simulink library "powerlib_models"  (Simulink 6.0)
settings: Solver=ode45  SolverMode=SingleTasking  StartTime=0.0  StopTime=10.0  RelTol=1e-3
values from neighbouring files (symbols this model uses):
  Ts = get(handles.edit1,'string')    [powergui.m]
undefined symbols (not defined in the file or in its folder): A, a0, a1, a2, a3, a4, a5, Ac, Amplitude, Amplitudes, B, BaseCurrent, BaseFlux, Bc, C, Capacitance, Cc, Columns, ConnectionType, Cs, ctrl, current, Current, damp, Dc, Dd, DiscIntNeverNeededParam, dref, dwo, exc, excAxis, F, Flux, fnom, Frequency, FreqVps, Gain1, gate, GH, GHd, GI, GId, GL, GLd, H, HarmonicGeneration, HT, hyd, I1_init, ib, ib2, Id1o, Inductance, InitialFlux, InitialSlope, io, Iq1o, isfinite, j, J ... (+138)
libraries: powerlib_models x32, powerlib_extras x4
(part 9 of 11)

== system powerlib_models/Phasors/simplified_sync_mach/Idq1 Idq2 Pe  ==
  note: I2= -V2/Z
  note: I1= (E-V1)/Z
  note: V1= 1/3(Vab -a^2*Vbc)
  note: V2= 1/3(Vab -a*Vbc)
  Vab Vbc cmplx : Inport  Port=1  LatchInput=off
  e : Inport  Port=2  LatchInput=off
  delta : Inport  Port=3  LatchInput=off
  (a^2)/3 : Gain  Gain=1/3*exp(-j*2*pi/3)  SaturateOnIntegerOverflow=on
  -1 : Gain  Gain=-1  SaturateOnIntegerOverflow=on
  1/Z1 : Gain  Gain=1/(R+j*L)  SaturateOnIntegerOverflow=on
  Complex to Real-Imag : ComplexToRealImag  Output=Real
  Complex to Real-Imag1 : ComplexToRealImag
  Complex to Real-Imag2 : ComplexToRealImag
  Complex to Real-Imag3 : ComplexToRealImag
  Demux : Demux  Outputs=2
  Gain : Gain  Gain=1/3  SaturateOnIntegerOverflow=on
  Gain1 : Gain  Gain=1/3  SaturateOnIntegerOverflow=on
  Magnitude-Angle to Complex1 : MagnitudeAngleToComplex
  Mux1 : Mux  Inputs=2
  Mux2 : Mux  Inputs=2
  Product : Product  SaturateOnIntegerOverflow=on  InputSameDT=on
  Real-Imag to Complex : RealImagToComplex
  Sum1 : Sum  Inputs=-+  SaturateOnIntegerOverflow=on  InputSameDT=on
  Sum3 : Sum  Inputs=+-  SaturateOnIntegerOverflow=on  InputSameDT=on
  Sum4 : Sum  Inputs=+-  SaturateOnIntegerOverflow=on  InputSameDT=on
  Vdq1->Idq1 : Subsystem
  Vdq2->Idq2 : Subsystem
  a/3 : Gain  Gain=1/3*exp(j*2*pi/3)  SaturateOnIntegerOverflow=on
  conj : Gain  Gain=-1  SaturateOnIntegerOverflow=on
  Pe : Outport
  Idq1 : Outport  Port=2
  Idq2 : Outport  Port=3
  wires:
  conj/1 -> Real-Imag to Complex/2
  Complex to Real-Imag1/2 -> conj/1
  Complex to Real-Imag1/1 -> Real-Imag to Complex/1
  Real-Imag to Complex/1 -> Product/2
  Magnitude-Angle to Complex1/1 -> Complex to Real-Imag1/1, Sum1/2  "E"
  Complex to Real-Imag/1 -> Pe/1
  Product/1 -> Complex to Real-Imag/1
  1/Z1/1 -> Product/1
  Sum1/1 -> 1/Z1/1, Complex to Real-Imag2/1  "U1=E1-V1"
  Sum3/1 -> Sum1/1  "V1"
  delta/1 -> Magnitude-Angle to Complex1/2
  e/1 -> Magnitude-Angle to Complex1/1
  Demux/1 -> Gain1/1, Gain/1
  a/3/1 -> Sum4/2
  Gain1/1 -> Sum4/1
  Vab Vbc cmplx/1 -> Demux/1
  Gain/1 -> Sum3/1
  Demux/2 -> a/3/1, (a^2)/3/1
  (a^2)/3/1 -> Sum3/2
  Sum4/1 -> -1/1  "V2"
  -1/1 -> Complex to Real-Imag3/1  "-V2"
  Complex to Real-Imag2/1 -> Mux1/1
  Complex to Real-Imag2/2 -> Mux1/2
  Complex to Real-Imag3/1 -> Mux2/1
  Complex to Real-Imag3/2 -> Mux2/2
  Mux1/1 -> Vdq1->Idq1/1(In1)
  Mux2/1 -> Vdq2->Idq2/1(In1)
  Vdq1->Idq1/1(Out1) -> Idq1/1
  Vdq2->Idq2/1(Out1) -> Idq2/1

== system powerlib_models/Phasors/simplified_sync_mach/LL2LN ==
  note: Vcn= -Van - Vbn
  note: Vbn=(Vbc - Vab)/3
  note: Van=(2*Vab+Vbc))/3
  Vab_bc : Inport  Port=1  LatchInput=off
  1/3 : Gain  Gain=1/3  SaturateOnIntegerOverflow=on
  2 : Gain  Gain=2  SaturateOnIntegerOverflow=on
  Demux : Demux  Outputs=2
  Mux2 : Mux  Inputs=3
  Sum1 : Sum  SaturateOnIntegerOverflow=on  InputSameDT=on
  Sum2 : Sum  Inputs=+-  SaturateOnIntegerOverflow=on  InputSameDT=on
  Sum6 : Sum  Orientation=down  Inputs=--  SaturateOnIntegerOverflow=on  InputSameDT=on
  Vabc_n : Outport
  wires:
  Demux/2 -> Sum2/1, Sum1/2
  2/1 -> Sum1/1
  Demux/1 -> Sum2/2, 2/1
  1/3/1 -> Demux/1
  Mux2/1 -> Vabc_n/1
  Vab_bc/1 -> 1/3/1
  Sum1/1 -> Sum6/2, Mux2/1  "Van"
  Sum2/1 -> Sum6/1, Mux2/2  "Vbn"
  Sum6/1 -> Mux2/3

== system powerlib_models/Phasors/simplified_sync_mach/Phasors Ia Ib ==
  note: Ib= a^2*I1 + a*I2
  note: Ia= I1 + I2
  Idq1 : Inport  Port=1  LatchInput=off
  Idq2 : Inport  Port=2  LatchInput=off
  Demux : Demux  Outputs=2
  Demux1 : Demux  Outputs=2
  Mux1 : Mux  Inputs=2
  Mux2 : Mux  Inputs=[2 1]
  Real-Imag to Complex : RealImagToComplex
  Real-Imag to Complex2 : RealImagToComplex
  Sum : Sum  Orientation=down  Inputs=1  SaturateOnIntegerOverflow=on  InputSameDT=on
  Sum1 : Sum  SaturateOnIntegerOverflow=on  InputSameDT=on
  Sum3 : Sum  SaturateOnIntegerOverflow=on  InputSameDT=on
  a : Gain  Gain=exp(j*2*pi/3)  SaturateOnIntegerOverflow=on
  a^2 : Gain  Gain=exp(-j*2*pi/3)  SaturateOnIntegerOverflow=on
  inv : Gain  Gain=-1  SaturateOnIntegerOverflow=on
  Iabc cmplx : Outport
  Iab cmplx : Outport  Port=2
  wires:
  Real-Imag to Complex2/1 -> a/1, Sum3/2  "I2"
  Idq2/1 -> Demux1/1
  Demux1/2 -> Real-Imag to Complex2/2
  Demux1/1 -> Real-Imag to Complex2/1
  Real-Imag to Complex/1 -> Sum3/1, a^2/1  "I1"
  Mux2/1 -> Iabc cmplx/1
  inv/1 -> Mux2/2  "ic"
  Sum/1 -> inv/1
  Mux1/1 -> Sum/1, Mux2/1, Iab cmplx/1  "ia ib"
  Demux/2 -> Real-Imag to Complex/2
  Demux/1 -> Real-Imag to Complex/1
  Idq1/1 -> Demux/1
  Sum1/1 -> Mux1/2
  Sum3/1 -> Mux1/1
  a/1 -> Sum1/2
  a^2/1 -> Sum1/1

== system powerlib_models/Phasors/simplified_sync_mach/Subsystem ==
  i : Inport  Port=1  LatchInput=off
  v : Inport  Port=2  LatchInput=off
  e : Inport  Port=3  LatchInput=off
  theta : Inport  Port=4  LatchInput=off
  wm : Inport  Port=5  LatchInput=off
  Pe : Inport  Port=6  LatchInput=off
  Gain : Gain  Gain=[ ib2*ones(3,1); Vb3*ones(6,1); 1; Nb; Pb ]  SaturateOnIntegerOverflow=on
  Mux : Mux  Inputs=[ 3 3 3 1 1 1 ]
  * : Outport  InitialOutput=0
  wires:
  Gain/1 -> */1
  Mux/1 -> Gain/1
  Pe/1 -> Mux/6
  wm/1 -> Mux/5
  theta/1 -> Mux/4
  e/1 -> Mux/3
  v/1 -> Mux/2
  i/1 -> Mux/1

== system powerlib_models/Phasors/synchronous_machine/Delta angle ==
  Vq : Inport  Port=1  PortDimensions=1  LatchInput=off
  Vd : Inport  Port=2  PortDimensions=1  LatchInput=off
  Cartesian to Polar : Subsystem
      mask Type: Cart2Polar
      mask Description:
      | Transformation from cartesian to polar coordinates.
      | [x, y] -> [r, theta]
      | 
      | r = sqrt(x^2 + y^2);
      | theta = atan(y/x);
      mask Help: Unmask this block for more help.
      mask Display: plot(0,0,100,100,[24,20,15,20,20],[85,95,85,95,20],[80,20,95,85,95,85],[70,20,20,15,20,24],[56,56,55,52,50,46],[20,26,31,35,38,42])
  Radians to Degrees : Subsystem
      mask Type: RadiansToDegrees
      mask Description:
      | Conversion from Radians to Degrees.
      | 
      | D=180/pi*R
      mask Help: This block converts from Radians to Degrees.
      mask Display: disp('R2D')
  Terminator2 : Terminator
  delta : Outport
  wires:
  Vd/1 -> Cartesian to Polar/2(y)
  Radians to Degrees/1(Degrees out) -> delta/1  "delta"
  Vq/1 -> Cartesian to Polar/1(x)
  Cartesian to Polar/1(r) -> Terminator2/1
  Cartesian to Polar/2(theta) -> Radians to Degrees/1(Radians in)

== system powerlib_models/Phasors/synchronous_machine/PQ ==
  note: P = Vd*Id + Vq*Iq
  note: Q = Vq*Id-Vd*Iq
  note: PQ Measurement:
  Vq : Inport  Port=1  PortDimensions=1  LatchInput=off
  Vd : Inport  Port=2  PortDimensions=1  LatchInput=off
  Iq : Inport  Port=3  PortDimensions=2  LatchInput=off
  Demux1 : Demux  Outputs=[1,1]
  Gain : Gain  Gain=Gain1  SaturateOnIntegerOverflow=on
  Gain1 : Gain  Gain=Gain1  SaturateOnIntegerOverflow=on
  Product{2..5} (4 alike) : Product  SaturateOnIntegerOverflow=on  InputSameDT=on
  Sum : Sum  SaturateOnIntegerOverflow=on  InputSameDT=on
  Sum1 : Sum  Inputs=+-  SaturateOnIntegerOverflow=on  InputSameDT=on
  Peo : Outport
  Qeo : Outport  Port=2
  wires:
  Demux1/1 -> Product5/2, Product2/2
  Iq/1 -> Demux1/1
  Gain1/1 -> Qeo/1
  Gain/1 -> Peo/1
  Product2/1 -> Sum/1
  Product3/1 -> Sum/2
  Product4/1 -> Sum1/1
  Product5/1 -> Sum1/2
  Sum/1 -> Gain/1  "Peo"
  Sum1/1 -> Gain1/1  "Qeo"
  Vd/1 -> Product3/1, Product5/1
  Vq/1 -> Product2/1, Product4/1
  Demux1/2 -> Product3/2, Product4/2

== system powerlib_models/Phasors/synchronous_machine/Phasors Ia Ib ==
  note: add angle d_theta
  note: Ib= a^2*I1 + a*I2
  note: Ia= I1 + I2
  Idq1 : Inport  Port=1  LatchInput=off
  d_theta : Inport  Port=2  LatchInput=off
  I2_cmplx : Inport  Port=3  LatchInput=off
  Demux : Demux  Outputs=2
  Gain2 : Gain  Gain=j  SaturateOnIntegerOverflow=on
  Math Function : Math  SaturateOnIntegerOverflow=on
  Mux1 : Mux  Inputs=2
  Mux2 : Mux  Inputs=[2 1]
  Product : Product  SaturateOnIntegerOverflow=on  InputSameDT=on
  Real-Imag to Complex : RealImagToComplex
  Sum : Sum  Orientation=down  Inputs=1  SaturateOnIntegerOverflow=on  InputSameDT=on
  Sum1 : Sum  SaturateOnIntegerOverflow=on  InputSameDT=on
  Sum3 : Sum  SaturateOnIntegerOverflow=on  InputSameDT=on
  a : Gain  Gain=exp(j*2*pi/3)  SaturateOnIntegerOverflow=on
  a^2 : Gain  Gain=exp(-j*2*pi/3)  SaturateOnIntegerOverflow=on
  inv : Gain  Gain=-1  SaturateOnIntegerOverflow=on
  Ia Ib cmplx : Outport
  Iabc cmplx : Outport  Port=2
  wires:
  d_theta/1 -> Gain2/1
  Real-Imag to Complex/1 -> Product/1  "I1 machine"
  Math Function/1 -> Product/2
  Gain2/1 -> Math Function/1
  Mux2/1 -> Iabc cmplx/1
  inv/1 -> Mux2/2  "ic"
  Sum/1 -> inv/1
  Mux1/1 -> Mux2/1, Ia Ib cmplx/1, Sum/1  "ia ib"
  Demux/2 -> Real-Imag to Complex/2
  Demux/1 -> Real-Imag to Complex/1
  Idq1/1 -> Demux/1
  Product/1 -> Sum3/1, a^2/1  "I1"
  Sum1/1 -> Mux1/2
  Sum3/1 -> Mux1/1
  a/1 -> Sum1/2
  a^2/1 -> Sum1/1
  I2_cmplx/1 -> Sum3/2, a/1  "I2"

== system powerlib_models/Phasors/synchronous_machine/Subsystem ==
  Vf : Inport  Port=1  LatchInput=off
  Constant : Constant  Value=excAxis
  Ground2 : Ground
  Switch : Switch  Threshold=1.5  InputSameDT=on
  Switch1 : Switch  Threshold=1.5  InputSameDT=on
  Vkq1 : Outport
  Vfd : Outport  Port=2
  wires:
  Switch/1 -> Vkq1/1
  Switch1/1 -> Vfd/1
  Constant/1 -> Switch1/2, Switch/2
  Vf/1 -> Switch/1, Switch1/3
  Ground2/1 -> Switch/3, Switch1/1

== system powerlib_models/Phasors/synchronous_machine/Vd1 Vq1, I2  ==
  note: Subtract angle d_theta
  note: V2= 1/3(Vab -a*Vbc)
  note: V1= 1/3(Vab -a^2*Vbc)
  Vab Vbc cmplx : Inport  Port=1  LatchInput=off
  d_theta : Inport  Port=2  LatchInput=off
  (a^2)/3 : Gain  Gain=1/3*exp(-j*2*pi/3)  SaturateOnIntegerOverflow=on
  Complex to Real-Imag1 : ComplexToRealImag
  Complex to Real-Imag2 : ComplexToRealImag
  Demux : Demux  Outputs=2
  Gain : Gain  Gain=1/3  SaturateOnIntegerOverflow=on
  Gain1 : Gain  Gain=1/3  SaturateOnIntegerOverflow=on
  Gain2 : Gain  Gain=-j  SaturateOnIntegerOverflow=on
  Math Function : Math  SaturateOnIntegerOverflow=on
  Mux2 : Mux  Inputs=2
  Product : Product  SaturateOnIntegerOverflow=on  InputSameDT=on
  Sum3 : Sum  Inputs=+-  SaturateOnIntegerOverflow=on  InputSameDT=on
  Sum4 : Sum  Inputs=+-  SaturateOnIntegerOverflow=on  InputSameDT=on
  Vdq2->Idq2 : Subsystem
  a/3 : Gain  Gain=1/3*exp(j*2*pi/3)  SaturateOnIntegerOverflow=on
  Vd : Outport
  Vq : Outport  Port=2
  I2_cmplx : Outport  Port=3
  wires:
  Math Function/1 -> Product/2
  Product/1 -> Complex to Real-Imag1/1
  Gain2/1 -> Math Function/1
  Sum4/1 -> Complex to Real-Imag2/1  "V2"
  (a^2)/3/1 -> Sum3/2
  Demux/2 -> (a^2)/3/1, a/3/1
  Complex to Real-Imag1/1 -> Vd/1
  Complex to Real-Imag1/2 -> Vq/1
  Sum3/1 -> Product/1  "V1"
  d_theta/1 -> Gain2/1
  Gain/1 -> Sum3/1
  Vab Vbc cmplx/1 -> Demux/1
  Gain1/1 -> Sum4/1
  a/3/1 -> Sum4/2
  Demux/1 -> Gain/1, Gain1/1
  Complex to Real-Imag2/1 -> Mux2/1
  Complex to Real-Imag2/2 -> Mux2/2
  Mux2/1 -> Vdq2->Idq2/1(V2_dq)
  Vdq2->Idq2/1(I2_cmplx) -> I2_cmplx/1

== system powerlib_models/Phasors/synchronous_machine/currents and mutual fluxes ==
  note: This subsystem computes the mutual fluxes phimd
      | and phimq and all direct and quadrature axis
      | currents in the model.
  phiq : Inport  Port=1  LatchInput=off
  phikq2 : Inport  Port=2  LatchInput=off
  phid : Inport  Port=3  LatchInput=off
  phifd : Inport  Port=4  LatchInput=off
  phikq1 : Inport  Port=5  LatchInput=off
  phikd : Inport  Port=6  LatchInput=off
  -1_Ll : Gain  Gain=-1/Ll  SaturateOnIntegerOverflow=on
  "-1_Ll " : Gain  Gain=-1/Ll  SaturateOnIntegerOverflow=on
  1_Llfd : Gain  Gain=1/Llfd  SaturateOnIntegerOverflow=on
  1_Llkd : Gain  Gain=1/Llkd  SaturateOnIntegerOverflow=on
  1_Llkq1 : Gain  Gain=1/Llkq1  SaturateOnIntegerOverflow=on
  1_Llkq2 : Gain  Gain=1/Llkq2  SaturateOnIntegerOverflow=on
  Lad_Ll : Gain  Gain=Lad/Ll  SaturateOnIntegerOverflow=on
  Lad_Llfd : Gain  Gain=Lad/Llfd  SaturateOnIntegerOverflow=on
  Lad_Llkd : Gain  Gain=Lad/Llkd  SaturateOnIntegerOverflow=on
  Laq_Ll : Gain  Gain=Laq/Ll  SaturateOnIntegerOverflow=on
  Laq_Llkq1 : Gain  Gain=Laq/Llkq1  SaturateOnIntegerOverflow=on
  Laq_Llkq2 : Gain  Gain=Laq/Llkq2  SaturateOnIntegerOverflow=on
  Mux1 : Mux  Inputs=2
  Mux3 : Mux  Inputs=[2 1 1 1 1 1 1]
  Saturation : Subsystem
  Sum{17..22} (6 alike) : Sum  Inputs=-+  SaturateOnIntegerOverflow=on  InputSameDT=on
  sum : Sum  Inputs=+++  SaturateOnIntegerOverflow=on  InputSameDT=on
  sum1 : Sum  Inputs=+++  SaturateOnIntegerOverflow=on  InputSameDT=on
  phimq : Outport  InitialOutput=0
  "iq,id,ifd, ikq1,ikq2,ikd, phimq,phimd" : Outport  Port=2  InitialOutput=0
  iq,id : Outport  Port=3  InitialOutput=0
  phimd : Outport  Port=4  InitialOutput=0
  wires:
  Saturation/2(phimd_out) -> Mux3/7, Sum19/1, Sum21/1, Sum20/1, phimd/1
  Saturation/1(phimq_out) -> Sum17/1, Mux3/6, Sum22/1, Sum18/1, phimq/1
  sum1/1 -> Saturation/2(phimd_in)  "phimd"
  sum/1 -> Saturation/1(phimq_in)  "phimq"
  Mux3/1 -> "iq,id,ifd, ikq1,ikq2,ikd, phimq,phimd"/1
  1_Llkq2/1 -> Mux3/4  "ikq2"
  1_Llkq1/1 -> Mux3/3  "ikq1"
  Sum20/1 -> "-1_Ll "/1
  "-1_Ll "/1 -> Mux1/2  "id"
  Sum21/1 -> 1_Llfd/1
  Sum19/1 -> 1_Llkd/1
  1_Llfd/1 -> Mux3/2  "ifd"
  1_Llkd/1 -> Mux3/5  "ikd"
  Sum18/1 -> 1_Llkq1/1
  Sum17/1 -> -1_Ll/1
  Sum22/1 -> 1_Llkq2/1
  -1_Ll/1 -> Mux1/1  "iq"
  Mux1/1 -> iq,id/1, Mux3/1
  Lad_Llkd/1 -> sum1/3
  Lad_Llfd/1 -> sum1/2
  Lad_Ll/1 -> sum1/1
  phifd/1 -> Lad_Llfd/1, Sum21/2
  phid/1 -> Sum20/2, Lad_Ll/1
  phikd/1 -> Lad_Llkd/1, Sum19/2
  phiq/1 -> Laq_Ll/1, Sum17/2
  Laq_Ll/1 -> sum/1
  Laq_Llkq2/1 -> sum/3
  Laq_Llkq1/1 -> sum/2
  phikq2/1 -> Laq_Llkq2/1, Sum22/2
  phikq1/1 -> Laq_Llkq1/1, Sum18/2

== system powerlib_models/Phasors/synchronous_machine/phid ==
  note: This subsystem computes the direct axis flux phid.
  w : Inport  Port=1  LatchInput=off
  phiq : Inport  Port=2  LatchInput=off
  vd : Inport  Port=3  LatchInput=off
  phimd : Inport  Port=4  LatchInput=off
  Product1 : Product  SaturateOnIntegerOverflow=on  InputSameDT=on
  Rs_Ll : Gain  Gain=Rs/Ll  SaturateOnIntegerOverflow=on
  Sum2 : Sum  Inputs=+++  SaturateOnIntegerOverflow=on  InputSameDT=on
  Sum9 : Sum  Inputs=+-  SaturateOnIntegerOverflow=on  InputSameDT=on
  int : Integrator  InitialCondition=phido
  web : Gain  Gain=web_psb  SaturateOnIntegerOverflow=on
  phid : Outport  InitialOutput=0
  wires:
  int/1 -> Sum9/2, phid/1
  web/1 -> int/1
  Sum2/1 -> web/1
  Rs_Ll/1 -> Sum2/3
  Sum9/1 -> Rs_Ll/1
  Product1/1 -> Sum2/1
  w/1 -> Product1/1
  phiq/1 -> Product1/2
  vd/1 -> Sum2/2
  phimd/1 -> Sum9/1

== system powerlib_models/Phasors/synchronous_machine/phifd ==
  note: This subsystem computes the field flux phifd.
  vfd : Inport  Port=1  LatchInput=off
  phimd : Inport  Port=2  LatchInput=off
  N : Gain  Gain=N  SaturateOnIntegerOverflow=on
  Rf_Llfd : Gain  Gain=Rf/Llfd  SaturateOnIntegerOverflow=on
  Sum10 : Sum  Inputs=+-  SaturateOnIntegerOverflow=on  InputSameDT=on
  Sum3 : Sum  SaturateOnIntegerOverflow=on  InputSameDT=on
  int : Integrator  InitialCondition=phifdo
  web : Gain  Gain=web_psb  SaturateOnIntegerOverflow=on
  phifd : Outport  InitialOutput=0
  wires:
  N/1 -> Sum3/1
  vfd/1 -> N/1
  Rf_Llfd/1 -> Sum3/2
  Sum10/1 -> Rf_Llfd/1
  phimd/1 -> Sum10/1
  web/1 -> int/1
  int/1 -> phifd/1, Sum10/2
  Sum3/1 -> web/1

== system powerlib_models/Phasors/synchronous_machine/phikd ==
  note: This subsystem computes the direct axis damper flux phikd.
  phimd : Inport  Port=1  LatchInput=off
  vkd : Inport  Port=2  LatchInput=off
  Rkd_Llkd : Gain  Gain=Rkd/Llkd  SaturateOnIntegerOverflow=on
  Sum11 : Sum  Inputs=-+  SaturateOnIntegerOverflow=on  InputSameDT=on
  Sum4 : Sum  SaturateOnIntegerOverflow=on  InputSameDT=on
  int : Integrator  InitialCondition=phikdo
  web : Gain  Gain=web_psb  SaturateOnIntegerOverflow=on
  phikd : Outport  InitialOutput=0
  wires:
  Rkd_Llkd/1 -> Sum4/1
  Sum11/1 -> Rkd_Llkd/1
  phimd/1 -> Sum11/2
  vkd/1 -> Sum4/2
  web/1 -> int/1
  int/1 -> phikd/1, Sum11/1
  Sum4/1 -> web/1

== system powerlib_models/Phasors/synchronous_machine/phikq1 ==
  note: This subsystem computes the quadrature axis damper flux phikq.
  phimq : Inport  Port=1  LatchInput=off
  vkq1 : Inport  Port=2  LatchInput=off
  Rkq1_Llkq1 : Gain  Gain=Rkq1/Llkq1  SaturateOnIntegerOverflow=on
  Sum1 : Sum  SaturateOnIntegerOverflow=on  InputSameDT=on
  Sum7 : Sum  Inputs=-+  SaturateOnIntegerOverflow=on  InputSameDT=on
  int : Integrator  InitialCondition=phikq1o
  web : Gain  Gain=web_psb  SaturateOnIntegerOverflow=on
  phikq1 : Outport  InitialOutput=0
  wires:
  int/1 -> Sum7/1, phikq1/1
  web/1 -> int/1
  vkq1/1 -> Sum1/2
  phimq/1 -> Sum7/2
  Sum1/1 -> web/1
  Sum7/1 -> Rkq1_Llkq1/1
  Rkq1_Llkq1/1 -> Sum1/1

== system powerlib_models/Phasors/synchronous_machine/phikq2 ==
  note: This subsystem computes the quadrature axis damper flux phikq2.
  vkq2 : Inport  Port=1  LatchInput=off
  phimq : Inport  Port=2  LatchInput=off
  Enabled integrator : Subsystem  TreatAsAtomicUnit=on
      mask Display: disp('1/s')
  Rkq2_Llkq2 : Gain  Gain=Rkq2/Llkq2  SaturateOnIntegerOverflow=on
  Sum1 : Sum  SaturateOnIntegerOverflow=on  InputSameDT=on
  Sum7 : Sum  Inputs=-+  SaturateOnIntegerOverflow=on  InputSameDT=on
  web : Gain  Gain=web_psb  SaturateOnIntegerOverflow=on
  wref : Constant  Value=isfinite(Llkq2)
  phikq2 : Outport  InitialOutput=0
  wires:
  wref/1 -> Enabled integrator/Enable
  Enabled integrator/1(Out1) -> phikq2/1, Sum7/1
  web/1 -> Enabled integrator/1(In1)
  Sum7/1 -> Rkq2_Llkq2/1
  vkq2/1 -> Sum1/2
  Rkq2_Llkq2/1 -> Sum1/1
  Sum1/1 -> web/1
  phimq/1 -> Sum7/2

== system powerlib_models/Phasors/synchronous_machine/phiq ==
  note: This subsystem computes the quadrature axis flux phiq.
  vq : Inport  Port=1  LatchInput=off
  w : Inport  Port=2  LatchInput=off
  phid : Inport  Port=3  LatchInput=off
  phimq : Inport  Port=4  LatchInput=off
  Product2 : Product  SaturateOnIntegerOverflow=on  InputSameDT=on
  Rs_Ll : Gain  Gain=Rs/Ll  SaturateOnIntegerOverflow=on
  Sum : Sum  Inputs=+-+  SaturateOnIntegerOverflow=on  InputSameDT=on
  Sum6 : Sum  Inputs=+-  SaturateOnIntegerOverflow=on  InputSameDT=on
  int1 : Integrator  InitialCondition=phiqo
  web : Gain  Gain=web_psb  SaturateOnIntegerOverflow=on
  phiq : Outport  InitialOutput=0
  wires:
  int1/1 -> Sum6/2, phiq/1
  web/1 -> int1/1
  phimq/1 -> Sum6/1
  phid/1 -> Product2/2
  w/1 -> Product2/1
  vq/1 -> Sum/1
  Product2/1 -> Sum/2
  Sum6/1 -> Rs_Ll/1
  Rs_Ll/1 -> Sum/3
  Sum/1 -> web/1

== system powerlib_models/Switch Current Source/IGBT/Conduction Logic ==
  iak : Inport  Port=1  LatchInput=off
  Vak : Inport  Port=2  LatchInput=off
  g : Inport  Port=3  LatchInput=off
  " " : RelationalOperator  Operator=>  InputSameDT=on
  "    " : Constant  Value=eps
  "      " : Constant  Value=0
  ". " : Logic
  . 1 : Logic  Operator=OR
  Break Alg. Loop : Subsystem  mask{Nsw=length(Ron)}
      mask prompts: Nsw "number of switches"
  Data Type  Conversion : DataTypeConversion  OutDataTypeMode=double  SaturateOnIntegerOverflow=on  RndMeth=Zero
  Data Type  Conversion1 : DataTypeConversion  OutDataTypeMode=double  SaturateOnIntegerOverflow=on  RndMeth=Zero
  Data Type  Conversion{2..3,5..6} (4 alike) : DataTypeConversion  OutDataTypeMode=boolean  SaturateOnIntegerOverflow=on  RndMeth=Zero
  Data Type  Conversion4 : DataTypeConversion  OutDataTypeMode=double  SaturateOnIntegerOverflow=on  RndMeth=Zero
  I>0 : Relay  OnSwitchValue=1000*eps  OffSwitchValue=0
  I>1.5 : Relay  OnSwitchValue=1.5  OffSwitchValue=0
  Test2 : Switch  Threshold=eps  InputSameDT=on
  Vf : Constant  Value=Vf
  b : RelationalOperator  Operator=>  InputSameDT=on
  n1 : Sum  SaturateOnIntegerOverflow=on  InputSameDT=on
  status : Outport  InitialOutput=0
  wires:
  Data Type  Conversion5/1 -> ". "/2, Test2/2
  Vak/1 -> b/1
  b/1 -> Data Type  Conversion6/1
  " "/1 -> Data Type  Conversion5/1
  Data Type  Conversion6/1 -> ". "/1
  g/1 -> Data Type  Conversion4/1
  Test2/1 -> status/1
  "      "/1 -> Test2/3  "zero current"
  Vf/1 -> b/2
  I>0/1 -> n1/1
  iak/1 -> I>0/1
  n1/1 -> I>1.5/1
  Data Type  Conversion/1 -> n1/2
  . 1/1 -> Data Type  Conversion1/1
  Data Type  Conversion1/1 -> Test2/1
  I>1.5/1 -> Data Type  Conversion2/1
  Data Type  Conversion2/1 -> . 1/1
  Data Type  Conversion3/1 -> . 1/2
  ". "/1 -> Break Alg. Loop/1(In1)
  Break Alg. Loop/1(Out1) -> Data Type  Conversion3/1, Data Type  Conversion/1
  Data Type  Conversion4/1 -> " "/1
  "    "/1 -> " "/2

== system powerlib_models/Switch Current Source/IGBT/Tail ==
  iak : Inport  Port=1  LatchInput=off
  switch : Inport  Port=2  LatchInput=off
  1 : Constant
  Integrator : Integrator  ExternalReset=falling  LimitOutput=on
  Look-Up  Table : Lookup  DialogController=Simulink.DDGSource  InputValues="[  0   Tf+eps Tf+Tt+2*eps  Tf+Tt+3*eps]"  OutputValues="[  1   0.1*(Tt>0) 0 0]"  SaturateOnIntegerOverflow=on
  Product : Product  SaturateOnIntegerOverflow=on  InputSameDT=on
  Switch : Switch  Threshold=eps  InputSameDT=on
  Iak : Outport  InitialOutput=0
  wires:
  Product/1 -> Switch/3
  Switch/1 -> Iak/1
  Integrator/1 -> Look-Up  Table/1
  1/1 -> Integrator/1
  switch/1 -> Integrator/2, Switch/2
  Look-Up  Table/1 -> Product/2
  iak/1 -> Switch/1, Product/1

== system powerlib_models/Switch Current Source/detailed_thyristor/Conduction logic ==
  Iak_meas. : Inport  Port=1  LatchInput=off
  Vak : Inport  Port=2  LatchInput=off
  G : Inport  Port=3  LatchInput=off
  "    " : Sum  Inputs=+++-  SaturateOnIntegerOverflow=on  InputSameDT=on
  ". " : Logic
  "0   " : Constant  Value=eps
  0.1 : Constant  Value=0.1
  Break Alg. Loop : Subsystem  mask{Nsw=length(Lon), IC=IC}
      mask prompts: Nsw "number of switches"; IC "initial conditions"
  Data Type  Conversion1 : DataTypeConversion  OutDataTypeMode=double  SaturateOnIntegerOverflow=on  RndMeth=Zero
  Data Type  Conversion3 : DataTypeConversion  OutDataTypeMode=double  SaturateOnIntegerOverflow=on  RndMeth=Zero
  Data Type  Conversion5 : DataTypeConversion  OutDataTypeMode=boolean  SaturateOnIntegerOverflow=on  RndMeth=Zero
  Data Type  Conversion6 : DataTypeConversion  OutDataTypeMode=boolean  SaturateOnIntegerOverflow=on  RndMeth=Zero
  I>1.5 : Relay  OnSwitchValue=1.5  OffSwitchValue=0
  Iak>IL : Relay  OnSwitchValue=eps+IL  OffSwitchValue=0
  Time recovery : Subsystem
  Vak>Vf : Subsystem
  b1 : RelationalOperator  Operator=>  InputSameDT=on
  n1 : Sum  SaturateOnIntegerOverflow=on  InputSameDT=on
  reset : Outport  InitialOutput=0
  wires:
  "0   "/1 -> b1/2
  Data Type  Conversion6/1 -> ". "/2
  b1/1 -> Data Type  Conversion6/1
  Data Type  Conversion5/1 -> ". "/1, Time recovery/2("Vak>Vf ")
  Vak>Vf/1(Vak>Vf) -> Data Type  Conversion5/1
  Data Type  Conversion3/1 -> b1/1
  G/1 -> Data Type  Conversion3/1
  Vak/1 -> Vak>Vf/1(Vak)
  Time recovery/1("TQ ") -> "    "/2
  0.1/1 -> "    "/4
  Iak_meas./1 -> Iak>IL/1
  Iak>IL/1 -> Time recovery/3(Iak>il), n1/1
  n1/1 -> I>1.5/1
  I>1.5/1 -> Time recovery/1(Iak>0), "    "/1
  "    "/1 -> Break Alg. Loop/1(In1)
  ". "/1 -> Data Type  Conversion1/1
  Data Type  Conversion1/1 -> "    "/3, n1/2
  Break Alg. Loop/1(Out1) -> reset/1

== system powerlib_models/Switch Current Source/detailed_thyristor/Switch-Ron-Lon ==
  Vak : Inport  Port=1  LatchInput=off
  Reset : Inport  Port=2  LatchInput=off
  "0 " : Constant  Orientation=left  Value=0
  "0   " : Constant  Orientation=left  Value=0
  Integrator : Integrator  ExternalReset=rising  InitialConditionSource=external
  L_device : Gain  Gain=1./Lon  SaturateOnIntegerOverflow=on
  R_device : Gain  Orientation=left  Gain=Ron  SaturateOnIntegerOverflow=on
  Step : Step  Orientation=left  Time=eps  Before=IC  After=0  SampleTime=0
  Test : Switch  Threshold=eps  InputSameDT=on
  Vak-Vf-Ron*Iak : Sum  Inputs=-+-  SaturateOnIntegerOverflow=on  InputSameDT=on
  Vf : Constant  Value=Vf
  test : Switch  Threshold=eps  InputSameDT=on
  "Iak  " : Outport  InitialOutput=0
  wires:
  "0 "/1 -> Test/3
  "0   "/1 -> test/3
  Step/1 -> Integrator/3
  Integrator/1 -> Test/1, R_device/1
  L_device/1 -> test/1
  test/1 -> Integrator/1
  Test/1 -> "Iak  "/1
  Vf/1 -> Vak-Vf-Ron*Iak/1
  Vak-Vf-Ron*Iak/1 -> L_device/1
  R_device/1 -> Vak-Vf-Ron*Iak/3
  Vak/1 -> Vak-Vf-Ron*Iak/2
  Reset/1 -> test/2, Integrator/2, Test/2

== system powerlib_models/Switch Current Source/diode/Conduction logic ==
  Iak : Inport  Port=1  LatchInput=off
  Vak : Inport  Port=2  LatchInput=off
  0 2 : Constant  Value=Vf
  0 3 : Constant  Value=0
  0 4 : Constant  Value=0
  Break Alg. Loop : Subsystem  AncestorBlock=powerlib_models/Switch Current Source/diode/Conduction logic/BAL-PB1  mask{Nsw=length(Lon), IC=IC}
      mask prompts: Nsw "number of switches"; IC "Initial condition"
  Data Type  Conversion1 : DataTypeConversion  OutDataTypeMode=boolean  SaturateOnIntegerOverflow=on  RndMeth=Zero
  Data Type  Conversion2 : DataTypeConversion  OutDataTypeMode=boolean  SaturateOnIntegerOverflow=on  RndMeth=Zero
  Data Type  Conversion3 : DataTypeConversion  OutDataTypeMode=boolean  SaturateOnIntegerOverflow=on  RndMeth=Zero
  b5 : RelationalOperator  Operator=>  InputSameDT=on
  b6 : RelationalOperator  Operator=>  InputSameDT=on
  b7 : RelationalOperator  Operator===  InputSameDT=on
  or2 : Logic  Operator=OR
  or3 : Logic
  status : Outport  InitialOutput=0
  wires:
  Vak/1 -> b6/1  "Vak diode"
  0 3/1 -> b7/2
  0 2/1 -> b6/2
  b6/1 -> Data Type  Conversion2/1  "Voltage > 0"
  or3/1 -> or2/2
  or2/1 -> Break Alg. Loop/1(In1)
  0 4/1 -> b5/2
  b5/1 -> Data Type  Conversion1/1  "Current > 0"
  b7/1 -> Data Type  Conversion3/1  "Current = 0"
  Iak/1 -> b5/1, b7/1  "Iak diode"
  Break Alg. Loop/1(Out1) -> status/1
  Data Type  Conversion1/1 -> or2/1
  Data Type  Conversion2/1 -> or3/1
  Data Type  Conversion3/1 -> or3/2

== system powerlib_models/Switch Current Source/gto/Conduction Logic ==
  iak : Inport  Port=1  LatchInput=off
  Vak : Inport  Port=2  LatchInput=off
  g : Inport  Port=3  LatchInput=off
  "      " : Constant  Value=0
  ". " : Logic
  . 1 : Logic  Operator=OR
  Break Alg. Loop : Subsystem  mask{Nsw=length(Ron)}
      mask prompts: Nsw "number of switches"
  Data Type  Conversion1 : DataTypeConversion  OutDataTypeMode=double  SaturateOnIntegerOverflow=on  RndMeth=Zero
  Data Type  Conversion{2..3,5..6} (4 alike) : DataTypeConversion  OutDataTypeMode=boolean  SaturateOnIntegerOverflow=on  RndMeth=Zero
  I>0 : Relay  OnSwitchValue=1000*eps  OffSwitchValue=0
  I>1.5 : Relay  OnSwitchValue=1.5  OffSwitchValue=0
  Test2 : Switch  Threshold=eps  InputSameDT=on
  Vf : Constant  Value=Vf
  b : RelationalOperator  Operator=>  InputSameDT=on
  n1 : Sum  SaturateOnIntegerOverflow=on  InputSameDT=on
  status : Outport  InitialOutput=0
  wires:
  Data Type  Conversion5/1 -> Test2/2, ". "/2
  Break Alg. Loop/1(Out1) -> Data Type  Conversion3/1, n1/2
  ". "/1 -> Break Alg. Loop/1(In1)
  Data Type  Conversion3/1 -> . 1/2
  Data Type  Conversion2/1 -> . 1/1
  I>1.5/1 -> Data Type  Conversion2/1
  Data Type  Conversion1/1 -> Test2/1
  . 1/1 -> Data Type  Conversion1/1
  n1/1 -> I>1.5/1
  iak/1 -> I>0/1
  I>0/1 -> n1/1
  Vf/1 -> b/2
  "      "/1 -> Test2/3
  Test2/1 -> status/1
  g/1 -> Data Type  Conversion5/1  "gate signal"
  Data Type  Conversion6/1 -> ". "/1
  b/1 -> Data Type  Conversion6/1
  Vak/1 -> b/1

== system powerlib_models/Switch Current Source/gto/Tail ==
  iak : Inport  Port=1  LatchInput=off
  switch : Inport  Port=2  LatchInput=off
  1 : Constant
  Integrator : Integrator  ExternalReset=falling  LimitOutput=on
  Look-Up  Table : Lookup  DialogController=Simulink.DDGSource  InputValues="[  0   Tf+eps Tf+Tt+2*eps  Tf+Tt+3*eps]"  OutputValues="[  1   0.1*(Tt>0) 0 0]"  SaturateOnIntegerOverflow=on
  Product : Product  SaturateOnIntegerOverflow=on  InputSameDT=on
  Switch : Switch  Threshold=eps  InputSameDT=on
  Iak : Outport  InitialOutput=0
  wires:
  iak/1 -> Product/1, Switch/1
  Look-Up  Table/1 -> Product/2
  switch/1 -> Switch/2, Integrator/2
  1/1 -> Integrator/1
  Integrator/1 -> Look-Up  Table/1
  Switch/1 -> Iak/1
  Product/1 -> Switch/3

== system powerlib_models/Switch Current Source/mosfet/Conduction Logic ==
  Ids_meas : Inport  Port=1  LatchInput=off
  Vds : Inport  Port=2  LatchInput=off
  G : Inport  Port=3  LatchInput=off
  "      1" : Constant
  . 1 : Logic  Operator=OR
  . 2 : Logic
  . 3 : Logic  Operator=NOT  Inputs=1
  Break Alg. Loop : Subsystem  mask{Nsw=length(Ron)}
      mask prompts: Nsw "number of switches"
  Data Type  Conversion : DataTypeConversion  OutDataTypeMode=double  SaturateOnIntegerOverflow=on  RndMeth=Zero
  Data Type  Conversion{1..2,4..5} (4 alike) : DataTypeConversion  OutDataTypeMode=boolean  SaturateOnIntegerOverflow=on  RndMeth=Zero
  Test2 : Switch  Threshold=eps  InputSameDT=on
  test_v : RelationalOperator  Operator=<  InputSameDT=on
  test_v1 : RelationalOperator  Operator=<  InputSameDT=on
  zero : Constant  Value=-eps
  zero1 : Constant  Value=-eps
  status : Outport  InitialOutput=0
  wires:
  Break Alg. Loop/1(Out1) -> Data Type  Conversion2/1
  "      1"/1 -> Test2/1
  Test2/1 -> status/1
  Data Type  Conversion/1 -> Test2/3
  test_v/1 -> Data Type  Conversion4/1
  Data Type  Conversion1/1 -> Test2/2, . 3/1
  Data Type  Conversion5/1 -> . 1/1
  test_v1/1 -> Data Type  Conversion5/1
  Data Type  Conversion4/1 -> . 2/1
  zero1/1 -> test_v1/2
  Ids_meas/1 -> test_v1/1
  zero/1 -> test_v/2
  . 2/1 -> Break Alg. Loop/1(In1)
  . 3/1 -> . 2/2
  . 1/1 -> Data Type  Conversion/1
  G/1 -> Data Type  Conversion1/1
  Vds/1 -> test_v/1
  Data Type  Conversion2/1 -> . 1/2

== system powerlib_models/Switch Current Source/thyristor/Conduction Logic ==
  "Iak " : Inport  Port=1  LatchInput=off
  Vak : Inport  Port=2  LatchInput=off
  "G " : Inport  Port=3  LatchInput=off
  0 1 : Constant  Value=0
  0 2 : Constant  Value=Vf
  0 3 : Constant  Value=0
  Break Alg. Loop : Subsystem  AncestorBlock=powerlib_models/Switch Current Source/thyristor/Conduction Logic/BAL-PB1  mask{Nsw=length(Lon), IC=IC}
      mask prompts: Nsw "number of switches"; IC "initial conditions"
  Data Type  Conversion{1..2,4,6} (4 alike) : DataTypeConversion  OutDataTypeMode=boolean  SaturateOnIntegerOverflow=on  RndMeth=Zero
  b5 : RelationalOperator  Operator=>  InputSameDT=on
  b6 : RelationalOperator  Operator=>  InputSameDT=on
  b7 : RelationalOperator  Operator===  InputSameDT=on
  or2 : Logic  Operator=OR
  or3 : Logic  Inputs=3
  Status : Outport  InitialOutput=0
  wires:
  Data Type  Conversion4/1 -> or3/3
  or3/1 -> or2/2
  or2/1 -> Break Alg. Loop/1(In1)
  b6/1 -> Data Type  Conversion2/1  "Voltage > Vf"
  b5/1 -> Data Type  Conversion1/1  "Current > 0"
  Vak/1 -> b6/1  "thyristor voltage"
  0 1/1 -> b5/2
  b7/1 -> Data Type  Conversion6/1  "Current = 0"
  0 3/1 -> b7/2
  0 2/1 -> b6/2
  "Iak "/1 -> b7/1, b5/1  "thyristor current"
  "G "/1 -> Data Type  Conversion4/1  "gate signal"
  Data Type  Conversion6/1 -> or3/2
  Data Type  Conversion1/1 -> or2/1
  Data Type  Conversion2/1 -> or3/1
  Break Alg. Loop/1(Out1) -> Status/1

== system powerlib_models/Continuous/Dynamic_Load/3-phase PLL1/2nd-Order Filter ==
  In : Inport  Port=1  LatchInput=off
  State-Space : StateSpace  A=Ac  B=Bc  C=Cc  D=Dc  X0=x0c
  Out : Outport  InitialOutput=0
  wires:
  State-Space/1 -> Out/1
  In/1 -> State-Space/1

== system powerlib_models/Continuous/Dynamic_Load/3-phase PLL1/Discrete PI Controller ==
  Error : Inport  Port=1  LatchInput=off
  Integrator : Integrator  InitialCondition=Init  LimitOutput=on  UpperSaturationLimit=UpperLimit  LowerSaturationLimit=LowerLimit
  Kp4 : Gain  Gain=Kp  SaturateOnIntegerOverflow=on
  Kp5 : Gain  Gain=Ki  SaturateOnIntegerOverflow=on
  Saturation2 : Saturate  UpperLimit=UpperLimit  LowerLimit=LowerLimit
  Sum6 : Sum  SaturateOnIntegerOverflow=on  InputSameDT=on
  Out : Outport  InitialOutput=0
  wires:
  Error/1 -> Kp4/1, Kp5/1
  Sum6/1 -> Saturation2/1
  Kp5/1 -> Integrator/1
  Kp4/1 -> Sum6/1
  Integrator/1 -> Sum6/2
  Saturation2/1 -> Out/1

== system powerlib_models/Continuous/Dynamic_Load/3-phase PLL1/Variable Frequency Mean value ==
  note: Mean Value (Variable frequency)
  note: Pierre Giroux, Gilbert Sybille
      | Power System Simulation Laboratory
      | IREQ, Hydro-Quebc
  Freq : Inport  Port=1  LatchInput=off
  In : Inport  Port=2  LatchInput=off
  Constant : Constant  Value=Vinit
  Integrator : Integrator
  Number of samples per cycle : Fcn  Expr=1/u[1]
  Product : Product  SaturateOnIntegerOverflow=on  InputSameDT=on
  Step : Step  Time=1/Finit  SampleTime=0
  Sum7 : Sum  Inputs=-+  SaturateOnIntegerOverflow=on  InputSameDT=on
  Switch : Switch  Threshold=0.5  InputSameDT=on
  To avoid division by zero : Saturate  Orientation=down  UpperLimit=1e6  LowerLimit=1e-6
  Variable Transport Delay : VariableTransportDelay  MaximumDelay=1/40  MaximumPoints=4096
  Mean : Outport
  wires:
  Number of samples per cycle/1 -> Variable Transport Delay/2  "Delay"
  Step/1 -> Switch/2
  To avoid division by zero/1 -> Number of samples per cycle/1  "Freq"
  Switch/1 -> Mean/1
  Constant/1 -> Switch/3
  Freq/1 -> To avoid division by zero/1, Product/2  "Freq"
  Integrator/1 -> Variable Transport Delay/1, Sum7/2
  Sum7/1 -> Product/1
  Variable Transport Delay/1 -> Sum7/1
  Product/1 -> Switch/1  "Mean value"
  In/1 -> Integrator/1  "In"

== system powerlib_models/Continuous/Dynamic_Load/3-phase PLL1/abc_to_dq1 ==
  note: This subsystem converts Vab and Vbc to Vd,Vq
  Vab_bc : Inport  Port=1  LatchInput=off
  sin_cos : Inport  Port=2  LatchInput=off
  Fcn2 : Fcn  Expr=(u[4]*(2*u[1]+u[2]) + (sqrt(3)*u[2]*u[3]))/3
  Fcn3 : Fcn  Expr=(u[3]*(2*u[1]+u[2]) + (-sqrt(3)*u[2]*u[4]))/3
  Mux1 : Mux  Inputs=[ 2 2 ]
  vd : Outport  InitialOutput=0
  vq : Outport  Port=2  InitialOutput=0
  wires:
  Vab_bc/1 -> Mux1/1
  Mux1/1 -> Fcn2/1, Fcn3/1
  sin_cos/1 -> Mux1/2
  Fcn2/1 -> vq/1
  Fcn3/1 -> vd/1

== system powerlib_models/Continuous/Dynamic_Load/Break  Alg. Loop/imag ==
  In1 : Inport  Port=1  LatchInput=off
  State Space : StateSpace  A=A  B=B  C=C  D=Dd  X0=X0
  Out1 : Outport  InitialOutput=0
  wires:
  In1/1 -> State Space/1
  State Space/1 -> Out1/1

== system powerlib_models/Continuous/Dynamic_Load/Break  Alg. Loop/real ==
  In1 : Inport  Port=1  LatchInput=off
  State Space : StateSpace  A=A  B=B  C=C  D=Dd  X0=X0
  Out1 : Outport  InitialOutput=0
  wires:
  In1/1 -> State Space/1
  State Space/1 -> Out1/1

== system powerlib_models/Continuous/Dynamic_Load/Positive Sequence  current/TF_P ==
  In1 : Inport  Port=1  LatchInput=off
  State-Space : StateSpace  A=Ac  B=Bc  C=Cc  D=Dc  X0=x0c
  Out1 : Outport
  wires:
  In1/1 -> State-Space/1
  State-Space/1 -> Out1/1

== system powerlib_models/Continuous/Dynamic_Load/Positive Sequence  current/TF_Q ==
  In1 : Inport  Port=1  LatchInput=off
  State-Space : StateSpace  A=Ac  B=Bc  C=Cc  D=Dc  X0=x0c
  Out1 : Outport
  wires:
  State-Space/1 -> Out1/1
  In1/1 -> State-Space/1

== system powerlib_models/Continuous/GTO-IGBT Bridge/Diode Logic/Blocking Diodes ==
  G : Inport  Port=1  LatchInput=off
  Bloque D214365 : Selector  Elements=Selec_Diode  InputPortWidth=nb_switch
  Logical Operator : Logic  Operator=NOT
  Memory : Memory  InheritSampleTime=on
  Pulse 1 step : Logic
  Block.D : Outport
  wires:
  Bloque D214365/1 -> Block.D/1
  Pulse 1 step/1 -> Bloque D214365/1  "Blockinkg"
  Memory/1 -> Logical Operator/1
  Logical Operator/1 -> Pulse 1 step/1
  G/1 -> Memory/1, Pulse 1 step/2

== system powerlib_models/Continuous/GTO-IGBT Bridge/Diode Logic/Trig.  Diodes (No Snubber Capacitance) ==
  G : Inport  Port=1  LatchInput=off
  Ipos : Inport  Port=2  LatchInput=off
  Enable : EnablePort  StatesWhenEnabling=reset
  Data Type  Conversion3 : DataTypeConversion  OutDataTypeMode=boolean  SaturateOnIntegerOverflow=on  RndMeth=Zero
  Logical Operator : Logic  Operator=NOT
  Memory : Memory  InheritSampleTime=on
  Pulse 1 step : Logic  Inputs=3
  Trig D214365 : Selector  Elements=Selec_Diode  InputPortWidth=nb_switch
  Trig D : Outport
  wires:
  Trig D214365/1 -> Trig D/1
  Pulse 1 step/1 -> Trig D214365/1
  Memory/1 -> Pulse 1 step/2
  Logical Operator/1 -> Pulse 1 step/1
  G/1 -> Memory/1, Logical Operator/1
  Ipos/1 -> Data Type  Conversion3/1
  Data Type  Conversion3/1 -> Pulse 1 step/3

== system powerlib_models/Continuous/MBPSS/Transfer function for detailed model (HF)/Transfer functions for detailed stabilizer ==
  In1 : Inport  Port=1  LatchInput=off
  Enable : EnablePort
  HF2 : TransferFcn  Numerator=[TH3 1]  Denominator=[TH4 1]
  HF3 : TransferFcn  Numerator=[TH5 1]  Denominator=[TH6 1]
  Out1 : Outport
  wires:
  In1/1 -> HF2/1
  HF3/1 -> Out1/1
  HF2/1 -> HF3/1

== system powerlib_models/Continuous/MBPSS/Transfer function for detailed model (HF)/Transfer functions for detailed stabilizer2 ==
  In1 : Inport  Port=1  LatchInput=off
  Enable : EnablePort
  HF5 : TransferFcn  Numerator=[TH9 1]  Denominator=[TH10 1]
  HF6 : TransferFcn  Numerator=[TH11 1]  Denominator=[TH12 1]
  Out1 : Outport
  wires:
  HF6/1 -> Out1/1
  In1/1 -> HF5/1
  HF5/1 -> HF6/1

== system powerlib_models/Continuous/MBPSS/Transfer function for detailed model (IF)/Transfer functions for detailed stabilizer ==
  In1 : Inport  Port=1  LatchInput=off
  Enable : EnablePort
  IF2 : TransferFcn  Numerator=[TI3 1]  Denominator=[TI4 1]
  IF3 : TransferFcn  Numerator=[TI5 1]  Denominator=[TI6 1]
  Out1 : Outport
  wires:
  IF3/1 -> Out1/1
  IF2/1 -> IF3/1
  In1/1 -> IF2/1

== system powerlib_models/Continuous/MBPSS/Transfer function for detailed model (IF)/Transfer functions for detailed stabilizer2 ==
  In1 : Inport  Port=1  LatchInput=off
  Enable : EnablePort
  IF5 : TransferFcn  Numerator=[TI9 1]  Denominator=[TI10 1]
  IF6 : TransferFcn  Numerator=[TI11 1]  Denominator=[TI12 1]
  Out1 : Outport
  wires:
  In1/1 -> IF5/1
  IF6/1 -> Out1/1
  IF5/1 -> IF6/1

== system powerlib_models/Continuous/MBPSS/Transfer function for detailed model (LF)/Transfer functions for detailed stabilizer ==
  In1 : Inport  Port=1  LatchInput=off
  Enable : EnablePort
  BF2 : TransferFcn  Numerator=[TL3 1]  Denominator=[TL4 1]
  BF3 : TransferFcn  Numerator=[TL5 1]  Denominator=[TL6 1]
  Out1 : Outport
  wires:
  BF2/1 -> BF3/1
  In1/1 -> BF2/1
  BF3/1 -> Out1/1

== system powerlib_models/Continuous/MBPSS/Transfer function for detailed model (LF)/Transfer functions for detailed stabilizer2 ==
  In1 : Inport  Port=1  LatchInput=off
  Enable : EnablePort
  BF5 : TransferFcn  Numerator=[TL9 1]  Denominator=[TL10 1]
  BF6 : TransferFcn  Numerator=[TL11 1]  Denominator=[TL12 1]
  Out1 : Outport
  wires:
  BF6/1 -> Out1/1
  In1/1 -> BF5/1
  BF5/1 -> BF6/1

== system powerlib_models/Continuous/PM_synchronous_machine/iq,id/id ==
  iq : Inport  Port=1  LatchInput=off
  we : Inport  Port=2  LatchInput=off
  vd : Inport  Port=3  LatchInput=off
  1/Ld : Gain  Gain=1/Ld  SaturateOnIntegerOverflow=on
  Lq/Ld : Gain  Gain=Lq/Ld  SaturateOnIntegerOverflow=on
  Product : Product  SaturateOnIntegerOverflow=on  InputSameDT=on
  R/Ld : Gain  Gain=R/Ld  SaturateOnIntegerOverflow=on
  Sum : Sum  Inputs=-++  SaturateOnIntegerOverflow=on  InputSameDT=on
  "id " : Integrator
  id : Outport  InitialOutput=0
  wires:
  1/Ld/1 -> Sum/2
  R/Ld/1 -> Sum/1
  Lq/Ld/1 -> Sum/3
  Sum/1 -> "id "/1
  Product/1 -> Lq/Ld/1
  "id "/1 -> R/Ld/1, id/1
  vd/1 -> 1/Ld/1
  we/1 -> Product/1
  iq/1 -> Product/2

== system powerlib_models/Continuous/PM_synchronous_machine/iq,id/iq ==
  vq : Inport  Port=1  LatchInput=off
  we : Inport  Port=2  LatchInput=off
  id : Inport  Port=3  LatchInput=off
  1/Lq : Gain  Gain=1/Lq  SaturateOnIntegerOverflow=on
  Ld/Lq : Gain  Gain=Ld/Lq  SaturateOnIntegerOverflow=on
  Product1 : Product  SaturateOnIntegerOverflow=on  InputSameDT=on
  R/Lq : Gain  Gain=R/Lq  SaturateOnIntegerOverflow=on
  Sum1 : Sum  Inputs=---+  SaturateOnIntegerOverflow=on  InputSameDT=on
  "iq " : Integrator
  lam/Lq : Gain  Gain=Flux/Lq  SaturateOnIntegerOverflow=on
  iq : Outport  InitialOutput=0
  wires:
  R/Lq/1 -> Sum1/1
  Ld/Lq/1 -> Sum1/2
  lam/Lq/1 -> Sum1/3
  Sum1/1 -> "iq "/1
  Product1/1 -> Ld/Lq/1
  1/Lq/1 -> Sum1/4
  id/1 -> Product1/1
  vq/1 -> 1/Lq/1
  we/1 -> Product1/2, lam/Lq/1
  "iq "/1 -> R/Lq/1, iq/1

== system powerlib_models/Continuous/Three-Level Bridge/2-level GTO-IGBT Bridge  Logic (modified)/Diode Logic ==
  Vak : Inport  Port=1  LatchInput=off
  G : Inport  Port=2  LatchInput=off
  0 2 : Constant  Value=0
  1 : Logic
  Blocking Diodes : Subsystem
  Data Type  Conversion5 : DataTypeConversion  OutDataTypeMode=boolean  SaturateOnIntegerOverflow=on  RndMeth=Zero
  Logical Operator3 : Logic  Operator=NOT
  b6 : RelationalOperator  Operator=>  InputSameDT=on
  status : Outport  InitialOutput=0
  block : Outport  Port=2  InitialOutput=0
  wires:
  Data Type  Conversion5/1 -> 1/1
  b6/1 -> Data Type  Conversion5/1
  Vak/1 -> b6/1
  0 2/1 -> b6/2
  G/1 -> Blocking Diodes/1(G)
  Blocking Diodes/1(Block.D) -> Logical Operator3/1, block/1
  Logical Operator3/1 -> 1/2
  1/1 -> status/1

== system powerlib_models/Continuous/Three-Level Bridge/2-level GTO-IGBT Bridge  Logic (modified)/GTO Logic ==
  Vak : Inport  Port=1  LatchInput=off
  G : Inport  Port=2  LatchInput=off
  " " : RelationalOperator  Operator=>  InputSameDT=on
  "    " : Constant  Value=0
  ". " : Logic
  Data Type  Conversion1 : DataTypeConversion  OutDataTypeMode=boolean  SaturateOnIntegerOverflow=on  RndMeth=Zero
  Data Type  Conversion2 : DataTypeConversion  OutDataTypeMode=boolean  SaturateOnIntegerOverflow=on  RndMeth=Zero
  Data Type  Conversion3 : DataTypeConversion  OutDataTypeMode=boolean  SaturateOnIntegerOverflow=on  RndMeth=Zero
  Vpos : Constant  Value=0
  b : RelationalOperator  Operator=>  InputSameDT=on
  status : Outport  InitialOutput=0
  wires:
  Data Type  Conversion3/1 -> " "/2
  "    "/1 -> Data Type  Conversion3/1
  Data Type  Conversion2/1 -> ". "/2
  " "/1 -> Data Type  Conversion2/1
  Data Type  Conversion1/1 -> ". "/1
  b/1 -> Data Type  Conversion1/1
  G/1 -> " "/1
  Vpos/1 -> b/2
  Vak/1 -> b/1
  ". "/1 -> status/1

== system powerlib_models/Continuous/Three-Level Bridge/2-level GTO-IGBT Bridge  Logic (modified)/Vf  ==
  status_GTO : Inport  Port=1  LatchInput=off
  Switch : Switch  Threshold=0.5  SaturateOnIntegerOverflow=on  InputSameDT=on
  Vf device : Constant  Value=Vf*ones(nb_switch,1)
  Vf diode : Constant  Value=-Vfd*ones(nb_switch,1)
  Vf : Outport  InitialOutput=[0]
  wires:
  Vf device/1 -> Switch/1
  Vf diode/1 -> Switch/3
  Switch/1 -> Vf/1
  status_GTO/1 -> Switch/2

== system powerlib_models/Continuous/Three-Level Bridge/Sw3 (clamping diode) Logic/Note 3 ==
  G : Inport  Port=1  LatchInput=off
  Logical Operator : Logic  Operator=NOT
  Memory : Memory
  Mux : Mux  Inputs=[nb_arm nb_arm]
  Pulse 1 step : Logic
  Select_BlockD : Selector  Elements=BlockDElements  InputPortWidth=nb_arm*2
  Block.D : Outport
  wires:
  Select_BlockD/1 -> Block.D/1
  Mux/1 -> Select_BlockD/1
  Pulse 1 step/1 -> Mux/1, Mux/2  "Blocking"
  G/1 -> Memory/1, Pulse 1 step/2
  Logical Operator/1 -> Pulse 1 step/1
  Memory/1 -> Logical Operator/1

== system powerlib_models/Continuous/Three-Level Bridge/Sw3 (clamping diode) Logic/Note 4 ==
  pulses : Inport  Port=1  LatchInput=off
  D5_On : Inport  Port=2  LatchInput=off
  D6_On : Inport  Port=3  LatchInput=off
  Status_GTO : Inport  Port=4  LatchInput=off
  Demux : Demux  Outputs=[nb_arm nb_arm nb_arm nb_arm]
  Demux1 : Demux  Outputs=[nb_arm nb_arm]
  Logical Operator{,4,6,10} (4 alike) : Logic  Operator=NOT
  Logical Operator1 : Logic  Operator=NOR  Inputs=4
  Logical Operator{2..3,5,9} (4 alike) : Logic  Inputs=3
  Logical Operator7 : Logic  Operator=OR
  Logical Operator8 : Logic  Operator=OR
  Memory{,1..3} (4 alike) : Memory
  Mux1 : Mux  Inputs=2
  Select_StatGTO : Selector  Elements=Trig12Elements  InputPortWidth=nb_arm*2
  Trig12 : Outport
  wires:
  Logical Operator9/1 -> Logical Operator7/2
  Logical Operator2/1 -> Logical Operator8/2
  Memory3/1 -> Logical Operator9/2
  Demux1/2 -> Memory3/1, Logical Operator10/1
  Logical Operator10/1 -> Logical Operator9/3
  Demux1/1 -> Memory2/1, Logical Operator6/1
  Select_StatGTO/1 -> Demux1/1
  Logical Operator8/1 -> Mux1/2
  Logical Operator5/1 -> Logical Operator8/1
  Logical Operator7/1 -> Mux1/1
  Logical Operator3/1 -> Logical Operator7/1
  Memory2/1 -> Logical Operator2/2
  Logical Operator6/1 -> Logical Operator2/3
  Status_GTO/1 -> Select_StatGTO/1
  Logical Operator1/1 -> Logical Operator9/1, Logical Operator2/1, Logical Operator5/1, Logical Operator3/3
  Demux/4 -> Logical Operator1/4
  Demux/3 -> Logical Operator1/3
  Demux/2 -> Logical Operator1/2
  Demux/1 -> Logical Operator1/1
  Mux1/1 -> Trig12/1
  Logical Operator4/1 -> Logical Operator5/3
  Memory1/1 -> Logical Operator5/2
  D5_On/1 -> Memory1/1, Logical Operator4/1
  Logical Operator/1 -> Logical Operator3/2
  Memory/1 -> Logical Operator3/1
  D6_On/1 -> Memory/1, Logical Operator/1
  pulses/1 -> Demux/1

== system powerlib_models/Continuous/Three-Level Bridge/Sw3 (clamping diode) Logic/Vf Computation for Sw3 ==
  D5_On : Inport  Port=1  LatchInput=off
  Gain1 : Gain  Gain=-1  SaturateOnIntegerOverflow=on
  Gain2 : Gain  SaturateOnIntegerOverflow=on
  Switch : Switch  Threshold=0.5  SaturateOnIntegerOverflow=on  InputSameDT=on
  Vf device : Constant  Value=(Vf+Vfd)*ones(nb_arm,1)
  Vf : Outport
  wires:
  Switch/1 -> Vf/1
  Vf device/1 -> Gain1/1, Gain2/1
  Gain1/1 -> Switch/1
  Gain2/1 -> Switch/3
  D5_On/1 -> Switch/2

== system powerlib_models/Continuous/asynchronous_machine/abc2qd/Rotor reference frame ==
  In1 : Inport  Port=1  LatchInput=off
  Enable : EnablePort  StatesWhenEnabling=reset
  Mux2 : Mux  Inputs=2
  Mux3 : Mux  Inputs=2
  vdr : Fcn  Expr=-sqrt3_3 * u[2]
  vds : Fcn  Expr=one_third * (2*u[5]*u[3] + (u[5]-sqrt3*u[6]) * u[4])
  vqr : Fcn  Expr=one_third * (2*u[1] + u[2])
  vqs : Fcn  Expr=one_third * (2*u[6]*u[3] + (u[6]+sqrt3*u[5]) * u[4])
  vqr,vdr : Outport  OutputWhenDisabled=reset  InitialOutput=0
  vqs,vds : Outport  Port=2  OutputWhenDisabled=reset  InitialOutput=0
  wires:
  vqs/1 -> Mux2/1
  vds/1 -> Mux2/2
  Mux2/1 -> vqs,vds/1  "Vqs,vds"
  vdr/1 -> Mux3/2
  vqr/1 -> Mux3/1
  Mux3/1 -> vqr,vdr/1  "Vqr,vdr"
  In1/1 -> vqr/1, vqs/1, vds/1, vdr/1

== system powerlib_models/Continuous/asynchronous_machine/abc2qd/Stationary reference frame ==
  In1 : Inport  Port=1  LatchInput=off
  Enable : EnablePort  StatesWhenEnabling=reset
  Mux2 : Mux  Inputs=2
  Mux3 : Mux  Inputs=2
  vdr : Fcn  Expr=one_third * (-2*u[5]*u[1] + (-u[5]-sqrt3*u[6]) * u[2])
  vds : Fcn  Expr=-sqrt3_3*u[4]
  vqr : Fcn  Expr=one_third * (2*u[6]*u[1] + (u[6]-sqrt3*u[5]) * u[2])
  vqs : Fcn  Expr=one_third * (2*u[3] + u[4])
  vqr,vdr : Outport  OutputWhenDisabled=reset  InitialOutput=0
  vqs,vds : Outport  Port=2  OutputWhenDisabled=reset  InitialOutput=0
  wires:
  vds/1 -> Mux2/2
  vqs/1 -> Mux2/1
  Mux2/1 -> vqs,vds/1  "Vqs,vds"
  vqr/1 -> Mux3/1
  vdr/1 -> Mux3/2
  In1/1 -> vqr/1, vds/1, vqs/1, vdr/1
  Mux3/1 -> vqr,vdr/1  "Vqr,vdr"

== system powerlib_models/Continuous/asynchronous_machine/abc2qd/Synchronous reference frame ==
  In1 : Inport  Port=1  LatchInput=off
  Enable : EnablePort  StatesWhenEnabling=reset
  Mux2 : Mux  Inputs=2
  Mux3 : Mux  Inputs=2
  vdr : Fcn  Expr=(2*u[5]*u[1] + (u[5]-sqrt3*u[6]) * u[2]) / 3
  vds : Fcn  Expr=(2*u[7]*u[3] + (u[7]-sqrt3*u[8]) * u[4]) / 3
  vqr : Fcn  Expr=(2*u[6]*u[1] + (u[6]+sqrt3*u[5]) * u[2]) / 3
  vqs : Fcn  Expr=(2*u[8]*u[3] + (u[8]+sqrt3*u[7]) * u[4]) / 3
  vqr,vdr : Outport  OutputWhenDisabled=reset  InitialOutput=0
  vqs,vds : Outport  Port=2  OutputWhenDisabled=reset  InitialOutput=0
  wires:
  vqs/1 -> Mux2/1
  vds/1 -> Mux2/2
  Mux2/1 -> vqs,vds/1  "Vqs,vds"
  vqr/1 -> Mux3/1
  vdr/1 -> Mux3/2
  In1/1 -> vqr/1, vds/1, vqs/1, vdr/1
  Mux3/1 -> vqr,vdr/1  "Vqr,vdr"

== system powerlib_models/Continuous/asynchronous_machine/abc2qd/transit ==
  vu : Inport  Port=1  LatchInput=off
  Constant6 : Constant  Value=[0;0]
  Mux1 : Mux  Inputs=2
  Selector : Selector  Elements=elements1  InputPortWidth=selWidth
  vr,vs : Outport
  wires:
  Constant6/1 -> Mux1/1
  Mux1/1 -> Selector/1
  vu/1 -> Mux1/2
  Selector/1 -> vr,vs/1

== system powerlib_models/Continuous/asynchronous_machine/dq2abc/Rotor reference frame ==
  In1 : Inport  Port=1  LatchInput=off
  Enable : EnablePort  StatesWhenEnabling=reset
  Mux1 : Mux  Inputs=2
  Mux2 : Mux  Inputs=2
  ira : Fcn  Expr=u[1]
  irb : Fcn  Expr=-(u[1] + sqrt3*u[2]) / 2
  isa : Fcn  Expr=u[6]*u[3]+u[5]*u[4]
  isb : Fcn  Expr=((-u[6]+sqrt3*u[5])*u[3] + (-sqrt3*u[6]-u[5])*u[4]) / 2
  ira,irb : Outport  OutputWhenDisabled=reset  InitialOutput=0
  isa,isb : Outport  Port=2  OutputWhenDisabled=reset  InitialOutput=0
  wires:
  ira/1 -> Mux1/1
  irb/1 -> Mux1/2
  isa/1 -> Mux2/1
  isb/1 -> Mux2/2
  In1/1 -> ira/1, irb/1, isa/1, isb/1
  Mux1/1 -> ira,irb/1  "ira,irb"
  Mux2/1 -> isa,isb/1  "isa,isb"
